simulink model "QuarkRefer"  (R2018a)
settings: Solver=FixedStepAuto  StartTime=0.0  StopTime=20  FixedStep=0.004  RelTol=1e-3
InitFcn:
  | seed1 = rand()*1000000;
  | seed2 = rand()*1000000;
  | seed3 = rand()*1000000;
libraries: quarc_library x4
settings Model: SimulationMode=external  ExtModeTrigDuration=5000  Creator=RSamra  LastModifiedBy=李玉玲
settings SolverCC: PositivePriorityOrder=on  AutoInsertRateTranBlk=on
settings DataIOCC: LimitDataPoints=on  SaveFormat=Array  SignalLoggingSaveFormat=ModelDataLogs  ReturnWorkspaceOutputs=on
settings OptimizationCC: ExpressionDepthLimit=2147483647  InitFltsAndDblsToZero=on  LifeSpan=inf
settings DebuggingCC: UnderspecifiedInitializationDetection=Classic  MergeDetectMultiDrivingBlocksExec=none  SolverPrmCheckMsg=warning  FcnCallInpInsideContextMsg=warning  StateNameClashWarn=warning  SFUnexpectedBacktrackingDiag=warning  SFNoUnconditionalDefaultTransitionDiag=warning  SFExecutionAtInitializationDiag=none
settings HardwareCC: ProdBitPerPointer=32  ProdBitPerSizeT=32  ProdBitPerPtrDiffT=32  ProdLargestAtomicFloat=None  ProdIntDivRoundTo=Undefined  ProdEndianess=Unspecified  ProdWordSize=32  ProdHWDeviceType=32-bit Generic
settings ModelReferenceCC: PropagateSignalLabelsOutOfModel=off
settings SFSimCC: SimParseCustomCode=off
settings RTWCC: SystemTargetFile=quarc_win64.tlc  TemplateMakefile=quarc_default_tmf  Description=QUARC Win64 Target
settings CodeAppCC: StateflowObjectComments=on
settings STFCustomTargetCC: TargetPreCompLibLocation=C:\PROGRA~3\QUARC\lib\2018a\win64\release  ConcurrentExecutionCompliant=on  CombineOutputUpdateFcns=on  CPPClassGenCompliant=on  GRTInterface=off  SystemTargetFile=quarc_win64.tlc
settings GRTTargetCC: TargetPreCompLibLocation=C:\PROGRA~3\QUARC\lib\2018a\win64\release  TargetLangStandard=C89/C90 (ANSI)  ParMdlRefBuildCompliant=off  CompOptLevelCompliant=off  MatFileLogging=off  UseToolchainInfoCompliant=off  ExtMode=on  ExtModeMexFile=quarc_comm
settings ConfigComp: CovMetricSettings=dw  CovSaveCumulativeToWorkspaceVar=on  CovSaveSingleToWorkspaceVar=on  CovExternalEMLEnable=off

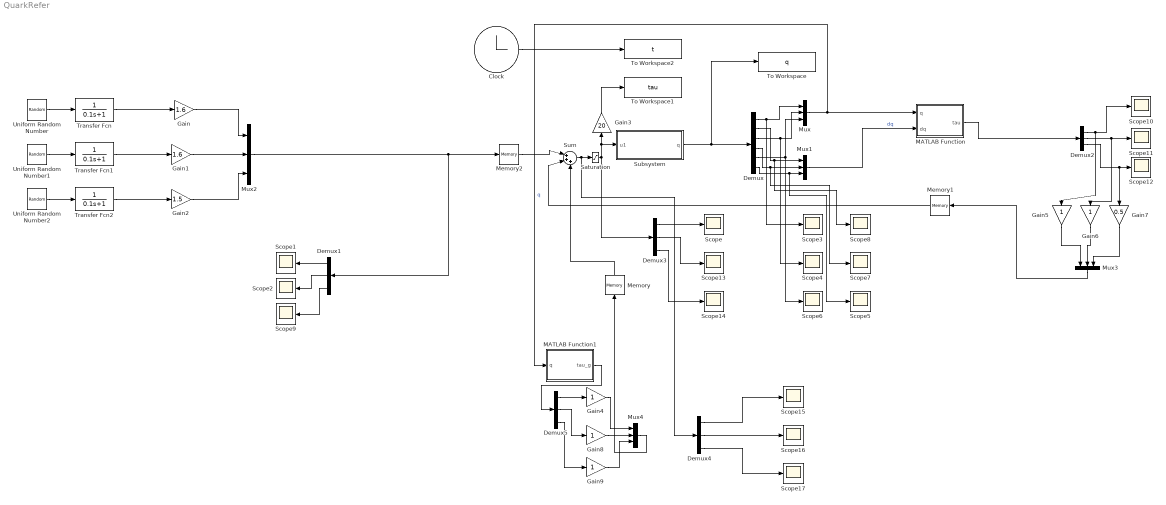
== system QuarkRefer ==
  Clock : Clock
      settings: Decimation=99999999
  Demux : Demux  Outputs=6
  Demux{1..5} (5 alike) : Demux  Outputs=3
  Gain : Gain  Gain=1.6
  Gain1 : Gain  Gain=1.6
  Gain2 : Gain  Gain=1.5
  Gain3 : Gain  Gain=20
  Gain{4..6,8..9} (5 alike) : Gain
  Gain7 : Gain  Gain=0.5
  MATLAB Function : MATLAB Function  TreatAsAtomicUnit=on
  MATLAB Function1 : MATLAB Function  TreatAsAtomicUnit=on
  Memory : quarc_library/Discrete/Memory  initial_condition=[0;0;0]  sample_time=-1
      settings: SourceProductName=QUARC Targets
  Memory1 : quarc_library/Discrete/Memory  initial_condition=0  sample_time=-1
      settings: SourceProductName=QUARC Targets
  Memory2 : quarc_library/Discrete/Memory  initial_condition=[0;0;0]  sample_time=-1
      settings: SourceProductName=QUARC Targets
  Mux{,1..4} (5 alike) : Mux  Inputs=3
  Saturation : Saturate  UpperLimit=[0.3 0.29 0.2]  LowerLimit=[-0.3 -0.29 -0.2]
  Scope{,1..17} (18 alike) : Scope
  Subsystem : Subsystem
  Sum : Sum  Inputs=|+++
  To Workspace : ToWorkspace  VariableName=q  SampleTime=-1
  To Workspace1 : ToWorkspace  VariableName=tau  SampleTime=-1
  To Workspace2 : ToWorkspace  VariableName=t  SampleTime=-1
  Transfer Fcn : TransferFcn  Denominator=[0.1 1]
  Transfer Fcn1 : TransferFcn  Denominator=[0.1 1]
  Transfer Fcn2 : TransferFcn  Denominator=[0.1 1]
  Uniform Random Number : UniformRandomNumber  Minimum=-0.3  Maximum=0.3  Seed=abs(seed1)  SampleTime=0.02
  Uniform Random Number1 : UniformRandomNumber  Minimum=-0.3  Maximum=0.3  Seed=abs(seed2)  SampleTime=0.02
  Uniform Random Number2 : UniformRandomNumber  Minimum=-0.2  Maximum=0.2  Seed=abs(seed3)  SampleTime=0.02
  wires:
  Gain1/1 -> Mux2/2
  Demux3/3 -> Scope14/1
  Transfer Fcn2/1 -> Gain2/1
  Clock/1 -> To Workspace2/1
  Uniform Random Number2/1 -> Transfer Fcn2/1
  Demux/2 -> Scope8/1, Mux1/1
  Sum/1 -> Demux4/1, Saturation/1
  Subsystem/1(q) -> To Workspace/1, Demux/1
  Demux3/2 -> Scope13/1
  Demux/4 -> Scope7/1, Mux1/2
  Transfer Fcn/1 -> Gain/1
  Mux2/1 -> Memory2/1, Demux1/1
  Demux1/3 -> Scope9/1
  Uniform Random Number/1 -> Transfer Fcn/1
  Saturation/1 -> Demux3/1, Subsystem/1(u1), Gain3/1
  Gain2/1 -> Mux2/3
  Uniform Random Number1/1 -> Transfer Fcn1/1
  Demux3/1 -> Scope/1
  Gain3/1 -> To Workspace1/1
  Demux2/3 -> Gain7/1, Scope12/1
  Mux1/1 -> MATLAB Function/2(dq)  "dq"
  Mux/1 -> MATLAB Function1/1(q), MATLAB Function/1(q)  "q"
  Demux/6 -> Scope5/1, Mux1/3
  Demux1/2 -> Scope2/1
  Demux2/2 -> Gain6/1, Scope11/1
  Memory1/1 -> Sum/2
  Demux/5 -> Scope6/1, Mux/3
  Memory/1 -> Sum/3
  Demux/3 -> Scope4/1, Mux/2
  Memory2/1 -> Sum/1
  Demux2/1 -> Gain5/1, Scope10/1
  Demux/1 -> Scope3/1, Mux/1
  MATLAB Function/1(tau) -> Demux2/1
  Gain/1 -> Mux2/1
  Transfer Fcn1/1 -> Gain1/1
  Demux1/1 -> Scope1/1
  MATLAB Function1/1(tau_g) -> Demux5/1
  Demux4/1 -> Scope15/1
  Demux4/2 -> Scope16/1
  Demux4/3 -> Scope17/1
  Gain5/1 -> Mux3/1
  Gain6/1 -> Mux3/2
  Gain7/1 -> Mux3/3
  Mux3/1 -> Memory1/1
  Demux5/1 -> Gain4/1
  Demux5/2 -> Gain8/1
  Demux5/3 -> Gain9/1
  Gain4/1 -> Mux4/1
  Gain8/1 -> Mux4/2
  Gain9/1 -> Mux4/3
  Mux4/1 -> Memory/1

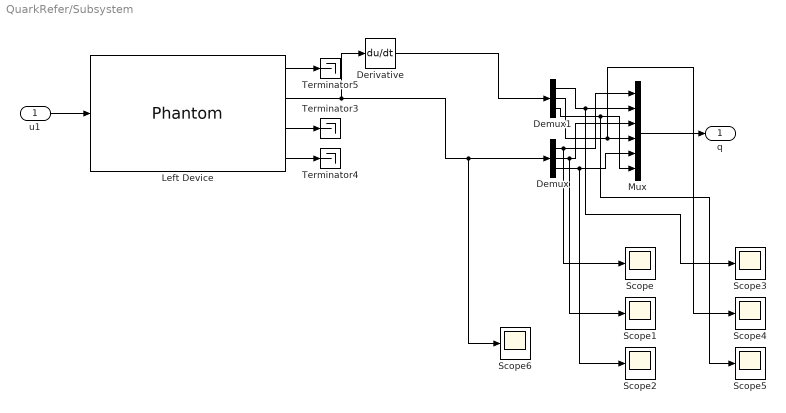
== system QuarkRefer/Subsystem ==
  u1 : Inport  PortDimensions=[3 1]
  Demux : Demux  Outputs=3
  Demux1 : Demux  Outputs=3
  Derivative : Derivative
  Left Device : quarc_library/Devices/Third-Party/SensAble/Phantom/Phantom  device_name=Default Device  output_type=Joint and Gimbal Angles  input_type=Joint space  velocity_limit_option=off  velocity_limit=1200  is_7dof=off  sample_time=0.004
      settings: AttributesFormatString=(%<device_name>)  SourceProductName=QUARC Targets
  Mux : Mux  Inputs=6
  Scope{,1..6} (7 alike) : Scope
  Terminator3 : Terminator
  Terminator4 : Terminator
  Terminator5 : Terminator
  q : Outport  PortDimensions=[6 1]
  wires:
  u1/1 -> Left Device/1
  Left Device/2 -> Scope6/1, Demux/1, Derivative/1
  Derivative/1 -> Demux1/1
  Left Device/3 -> Terminator3/1
  Left Device/4 -> Terminator4/1
  Left Device/1 -> Terminator5/1
  Demux/1 -> Scope/1, Mux/1
  Demux/2 -> Scope1/1, Mux/3
  Demux/3 -> Scope2/1, Mux/5
  Demux1/1 -> Scope3/1, Mux/2
  Demux1/2 -> Scope4/1, Mux/4
  Demux1/3 -> Scope5/1, Mux/6
  Mux/1 -> q/1

== matlab function QuarkRefer/MATLAB Function1 ==
  data: q input; tau_g output
function tau_g = gravity_comp(q)
% GRAVITY_COMP 计算 robot2 模型的重力补偿力矩
% 输入:
%   q - 关节位置向量 [q1, q2, q3] (可以是行向量或列向量)
% 输出:
%   tau_g - 重力补偿力矩向量 [tau_g1, tau_g2, tau_g3]

    % --- 模型参数 (来自 robot2.m) ---
    % p = [p1, p2, p3, p4, p5, p6, p7, p8, p9]
    p = [3.7*10^(-3) 7*10^(-3) 8*10^(-3) 0.4*10^(-3) 9.1*10^(-3) 5.2*10^(-3) 0.096 0.145 0.055];
    g = 9.8; % 重力加速度

    % --- 提取关节位置 ---
    % 假设 q 输入为 [q1, q2, q3]
    % q1 = q(1); % 关节1位置 (对重力无影响)
    q2 = q(2);   % 关节2位置 (对应 robot2 中的 x(3))
    q3 = q(3);   % 关节3位置 (对应 robot2 中的 x(5))

    % --- 计算重力项 G(q) ---
    % G1 = 0
    % G2 = p(5)*g*cos(q2) + p(6)*g*cos(q2+q3)
    % G3 = p(6)*g*cos(q2+q3)
    
    tau_g1 = 0;
    tau_g2 = p(5) * g * cos(q2) + p(6) * g * cos(q2 + q3);
    tau_g3 = p(6) * g * cos(q2 + q3);

    % --- 构造输出向量 ---
    tau_g = [tau_g1; tau_g2; tau_g3];
    
end

== matlab function QuarkRefer/MATLAB Function ==
  data: q input; tau output; dq input
function tau = fcn(q,dq)
% 读取输入
q1 = q(1); q2 = q(2); q3 = q(3);
dq1 = dq(1); dq2 = dq(2); dq3 = dq(3);

% --- 1. 定义参数 ---
k = 4;      % 非线性刚度的指数 (越大约“陡峭”)
K = [0.5, 0.5, 0.5]; % [K1, K2, K3] 最大刚度系数
A = [0.01, 0.01, 0.01]; % [A1, A2, A3] 阻尼系数

% --- 2. 定义每个关节的运动范围 [min, max] ---
% 关节1: [-pi/3, pi/3]
q1_min = -pi/3;  q1_max = pi/3;
% 关节2: [0, 1.79]
q2_min = 0.27;      q2_max = 2.0;
% 关节3: [-2.45, -0.25]
q3_min = -0.14;  q3_max = 1.95;

% --- 3. 计算中心点 (Target) 和 半宽度 (Scale) ---
q1_ctr = (q1_min + q1_max) / 2;  L1 = (q1_max - q1_min) / 2;
q2_ctr = (q2_min + q2_max) / 2;  L2 = (q2_max - q2_min) / 2;
q3_ctr = (q3_min + q3_max) / 2;  L3 = (q3_max - q3_min) / 2;

% --- 4. 计算位置误差 (Error = current - target) ---
% 注意：您原来的 -q1 实际上是 (0 - q1)，即 (target - current)
% 这里为了和物理意义一致，我们定义 error = q - q_ctr (当前 - 目标)
% 那么恢复力方向就是负的： - error
err1 = q1 - q1_ctr;
err2 = q2 - q2_ctr;
err3 = q3 - q3_ctr;

% --- 5. 计算势能整形力矩 (Position Term) ---
% 原公式: tau = (abs(q)/(pi/2))^k * K * (-q)
% 新公式: tau = (abs(err)/L)^k * K * (-err)
% 解析:
% - (abs(err)/L)^k : 归一化的非线性增益系数。在中心为0，在边界为1。
% - K             : 全局刚度放大系数。
% - (-err)        : 线性恢复力部分，包含了方向(指向中心)和幅值(距离中心的绝对距离)。

tau1_p = (abs(err1) / L1)^k * K(1) * (-err1);
tau2_p = (abs(err2) / L2)^k * K(2) * (-err2);
tau3_p = (abs(err3) / L3)^k * K(3) * (-err3);

% --- 6. 计算阻尼力矩 (Velocity Term) ---
tau1_d = A(1) * (-dq1);
tau2_d = A(2) * (-dq2);
tau3_d = A(3) * (-dq3);

% --- 7. 总输出力矩 ---
tau = [tau1_p + tau1_d; tau2_p + tau2_d; tau3_p + tau3_d];

end
